simulink model "readGyroscope"  (R2019a)
settings: Solver=FixedStepAuto  StartTime=0.0  StopTime=inf  RelTol=1e-3  EnableMultiTasking=on
libraries: raspberrypilib x3, simulink x1
settings Model: SimulationMode=external  Creator=florian  LastModifiedBy=christinefux
settings SolverCC: PositivePriorityOrder=on
settings OptimizationCC: EnhancedBackFolding=on  PassReuseOutputArgsAs=Individual arguments  MaxStackSize=64  OptimizeBlockOrder=speed  DifferentSizesBufferReuse=on  OptimizationCustomize=off
settings DebuggingCC: ParameterTunabilityLossMsg=error
settings HardwareCC: ProdBitPerPointer=32  ProdBitPerSizeT=32  ProdBitPerPtrDiffT=32  ProdLargestAtomicInteger=Long  ProdLargestAtomicFloat=Double  ProdWordSize=32  ProdLongLongMode=on  ProdHWDeviceType=ARM Compatible->ARM Cortex
settings SFSimCC: MATLABDynamicMemAlloc=off
settings RTWCC: SystemTargetFile=ert.tlc  HardwareBoard=Raspberry Pi  TLCOptions="-aInlineSetEventsForThisBaseRateFcn=TLC_FALSE -aSuppressMultiTaskScheduler=TLC_FALSE  -aRateBasedStepFcn=0"  TemplateMakefile=ert_default_tmf  GenerateReport=on  Toolchain=GNU GCC Raspberry Pi  BuildConfiguration=Faster Runs  IncludeHyperlinkInReport=on  LaunchReport=on  GenerateTraceInfo=on  GenerateTraceReport=on  GenerateTraceReportSl=on  GenerateTraceReportSf=on  GenerateTraceReportEml=on
settings CodeAppCC: ForceParamTrailComments=on  IgnoreCustomStorageClasses=off  OperatorAnnotations=on  SimulinkDataObjDesc=on  SFDataObjDesc=on  InsertBlockDesc=on
settings ERTTargetCC: SupportContinuousTime=on  SupportVariableSizeSignals=on

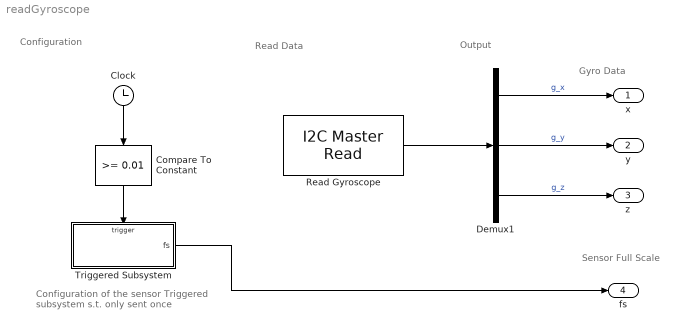
== system readGyroscope ==
  note: Configuration
  note: Configuration of the sensor
      | Triggered subsystem s.t. only sent once
  note: Read Data
  note: Output
  note: Gyro Data
  note: Sensor Full Scale
  Clock : Clock
  Compare To Constant : simulink/Logic and Bit Operations/Compare To Constant  relop=>=  const=0.01  OutDataTypeStr=boolean
  Demux1 : Demux  Outputs=3
  Read Gyroscope : raspberrypilib/I2C Master Read  Priority=1  BoardProperty=Pi 3 Model B+  Mode=Master  SlaveAddress=107  SlaveByteOrder=LittleEndian  Direction=Receiver  RegisterAddressMode=on  RegisterAddress=34  SlaveDataType=int16  DataLength=3  NoAck=off  RepeatedStart=off  OutputStatus=off  SampleTime=8.0E-5
      settings: SourceProductName=Simulink Support Package for Raspberry Pi Hardware  SourceProductBaseCode=RASPPI
  Triggered Subsystem : Subsystem  TreatAsAtomicUnit=on
  x : Outport
  y : Outport  Port=2
  z : Outport  Port=3
  fs : Outport  Port=4
  wires:
  Demux1/2 -> y/1  "g_y"
  Demux1/1 -> x/1  "g_x"
  Read Gyroscope/1 -> Demux1/1
  Demux1/3 -> z/1  "g_z"
  Compare To Constant/1 -> Triggered Subsystem/Trigger
  Clock/1 -> Compare To Constant/1
  Triggered Subsystem/1(fs) -> fs/1

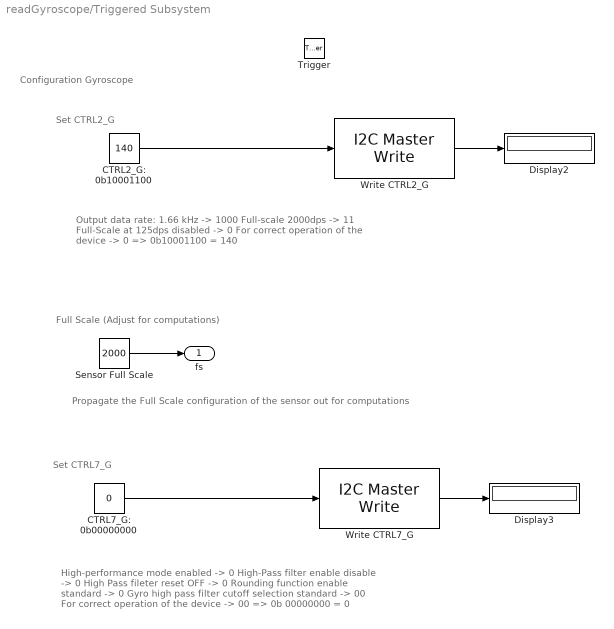
== system readGyroscope/Triggered Subsystem ==
  note: Configuration Gyroscope
  note: Propagate the Full Scale configuration of the sensor out for computations
  note: Full Scale (Adjust for computations)
  note: Output data rate:				 	1.66 kHz		-> 1000
      | Full-scale						2000dps		-> 11
      | Full-Scale at 125dps				disabled		-> 0
      | For correct operation of the device				-> 0
      | 								=> 0b10001100 = 140
  note: High-performance mode				enabled			-> 0
      | High-Pass filter enable				disable			-> 0
      | High Pass fileter reset					OFF			-> 0
      | Rounding function enable				standard			-> 0
      | Gyro high pass filter cutoff selection		standard			-> 00
      | For correct operation of the device						-> 00
      | 									=> 0b 00000000 = 0
  note: Set CTRL2_G
  note: Set CTRL7_G
  Trigger : TriggerPort  VariantControl=Variant
  CTRL2_G: 0b10001100 : Constant  Value=140  OutDataTypeStr=uint8
  CTRL7_G: 0b00000000 : Constant  Value=0  OutDataTypeStr=uint8
  Display2 : Display
  Display3 : Display
  Sensor Full Scale : Constant  Value=2000
  Write CTRL2_G : raspberrypilib/I2C Master Write  Priority=0  BoardProperty=Pi 3 Model B+  Mode=Master  SlaveAddress=107  SlaveByteOrder=LittleEndian  Direction=Transmitter  RegisterAddressMode=on  RegisterAddress=17  SlaveDataType=uint8  DataLength=1  NoAck=off  RepeatedStart=off  OutputStatus=on
      settings: SourceProductName=Simulink Support Package for Raspberry Pi Hardware  SourceProductBaseCode=RASPPI
  Write CTRL7_G : raspberrypilib/I2C Master Write  Priority=0  BoardProperty=Pi 3 Model B+  Mode=Master  SlaveAddress=107  SlaveByteOrder=LittleEndian  Direction=Transmitter  RegisterAddressMode=on  RegisterAddress=22  SlaveDataType=uint8  DataLength=1  NoAck=off  RepeatedStart=off  OutputStatus=on
      settings: SourceProductName=Simulink Support Package for Raspberry Pi Hardware  SourceProductBaseCode=RASPPI
  fs : Outport
  wires:
  CTRL7_G: 0b00000000/1 -> Write CTRL7_G/1
  CTRL2_G: 0b10001100/1 -> Write CTRL2_G/1
  Write CTRL2_G/1 -> Display2/1
  Write CTRL7_G/1 -> Display3/1
  Sensor Full Scale/1 -> fs/1
